simulink subsystem "anode_subsystem_humidification"  (R2023a)
settings: Solver=VariableStepAuto  StartTime=0.0  StopTime=10.0  RelTol=1e-3
settings Model: Creator=stefan.notter  LastModifiedBy=stefan.notter

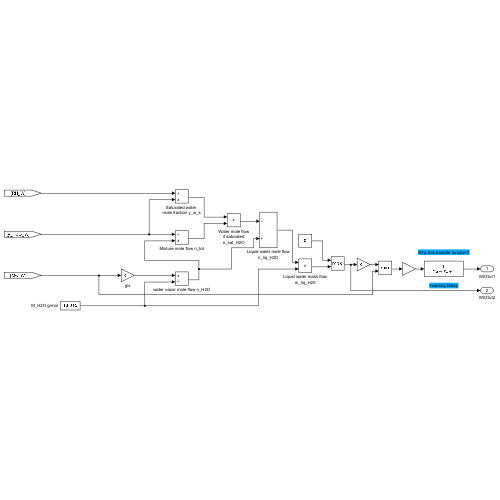
[thumbnail: Simulink's stored preview of the top-level diagram]
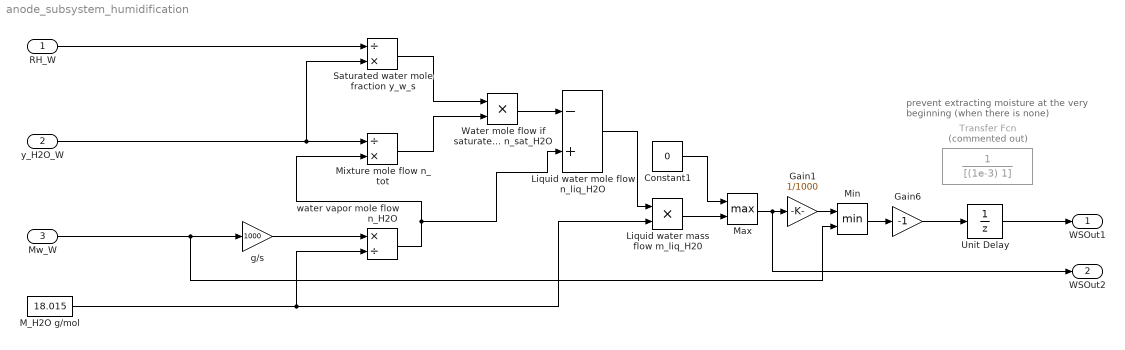
== system anode_subsystem_humidification ==
  note: prevent extracting moisture at the very beginning (when there is none)
  RH_W : Inport
  y_H2O_W : Inport  Port=2
  Mw_W : Inport  Port=3
  Constant1 : Constant  Value=0
  Gain1 : Gain  Gain=1/1000
  Gain6 : Gain  Gain=-1
  Liquid water mass flow m_liq_H20 : Product
  Liquid water mole flow n_liq_H2O : Sum  Inputs=-+
  M_H2O g/mol : Constant  Value=18.015
  Max : MinMax  Function=max  Inputs=2
  Min : MinMax  Inputs=2
  Mixture mole flow n_tot : Product  Inputs=/*
  Saturated water mole fraction y_w_s : Product  Inputs=/*
  Transfer Fcn : TransferFcn  Commented=on  Denominator=[(1e-3) 1]
  Unit Delay : UnitDelay  SampleTime=-1  HasFrameUpgradeWarning=on
  Water mole flow if saturated n_sat_H2O : Product
  g/s : Gain  Gain=1000
  water vapor mole flow n_H2O : Product  Inputs=*/
  WSOut1 : Outport
  WSOut2 : Outport  Port=2
  wires:
  Constant1/1 -> Max/1
  Unit Delay/1 -> WSOut1/1
  Gain1/1 -> Min/1
  Liquid water mass flow m_liq_H20/1 -> Max/2
  Water mole flow if saturated n_sat_H2O/1 -> Liquid water mole flow n_liq_H2O/1
  Gain6/1 -> Unit Delay/1
  Liquid water mole flow n_liq_H2O/1 -> Liquid water mass flow m_liq_H20/1
  Mixture mole flow n_tot/1 -> Water mole flow if saturated n_sat_H2O/2
  Saturated water mole fraction y_w_s/1 -> Water mole flow if saturated n_sat_H2O/1
  water vapor mole flow n_H2O/1 -> Liquid water mole flow n_liq_H2O/2, Mixture mole flow n_tot/2
  M_H2O g/mol/1 -> water vapor mole flow n_H2O/2, Liquid water mass flow m_liq_H20/2
  Max/1 -> WSOut2/1, Gain1/1
  g/s/1 -> water vapor mole flow n_H2O/1
  Min/1 -> Gain6/1
  Mw_W/1 -> g/s/1, Min/2
  RH_W/1 -> Saturated water mole fraction y_w_s/1
  y_H2O_W/1 -> Saturated water mole fraction y_w_s/2, Mixture mole flow n_tot/1
